simulink model "rl_distillation"  (R2022b)
settings: Solver=ode45  StartTime=0.0  StopTime=Tf  RelTol=1e-3  EnableMultiTasking=on
model workspace (MAT data in the model file):
  DM0 = [1  0; 0  1]
  G = tf
  G.InputName_ = ["u1"; "u2"]
  G.OutputName_ = ["y1"; "y2"]
  G.IOSize_ = [2 2]
  G.Data_ = ltipack.tfdata
  G.Data_.num = {[0 87.8], [0 -86.4]; [0 108.2], [0 -109.6]}
  G.Data_.den = {[75 1], [75 1]; [75 1], [75 1]}
  G.Data_.Delay.Input = [0; 0]
  G.Data_.Delay.Output = [0; 0]
  G.Data_.Delay.IO = [0  0; 0  0]
  G.Data_.Ts = 0
undefined symbols (not defined in the file or in its folder): random_refs_table, Tf
libraries: slpidlib x2, cstblocks x1, rllib x1
settings Model: Creator=The MathWorks, Inc.  LastModifiedBy=enes
settings SolverCC: AlgebraicLoopSolver=TrustRegion  MaxZcPerStep=1
settings DataIOCC: LimitDataPoints=on  SaveFormat=Array  ReturnWorkspaceOutputs=off
settings OptimizationCC: ExpressionDepthLimit=2147483647  LifeSpan=inf
settings DebuggingCC: UnderspecifiedInitializationDetection=Classic  MergeDetectMultiDrivingBlocksExec=none  FcnCallInpInsideContextMsg=warning  UnconnectedInputMsg=warning  UnconnectedOutputMsg=warning  UnconnectedLineMsg=warning  StateNameClashWarn=warning  SFUnexpectedBacktrackingDiag=warning  SFNoUnconditionalDefaultTransitionDiag=warning  SFMachineParentedDataDiag=warning  ArithmeticOperatorsInVariantConditions=warning
settings HardwareCC: ProdBitPerPointer=32  ProdBitPerSizeT=32  ProdBitPerPtrDiffT=32  ProdLargestAtomicFloat=None  ProdIntDivRoundTo=Undefined  ProdEndianess=Unspecified  ProdWordSize=32  ProdHWDeviceType=32-bit Generic
settings ModelReferenceCC: EnableRefExpFcnMdlSchedulingChecks=on  PropagateSignalLabelsOutOfModel=off
settings SFSimCC: SimUseLocalCustomCode=off  CustomCodeUndefinedFunction=UseInterfaceOnly
settings RTWCC: RTWUseLocalCustomCode=off  DLArmComputeVersion=19.05
settings CodeAppCC: StateflowObjectComments=on
settings GRTTargetCC: TargetLangStandard=C89/C90 (ANSI)  CombineOutputUpdateFcns=off  GRTInterface=on
settings ConfigComp: CovMetricSettings=dw  CovSaveCumulativeToWorkspaceVar=on  CovSaveSingleToWorkspaceVar=on  CovExternalEMLEnable=off  CovSFcnEnable=off

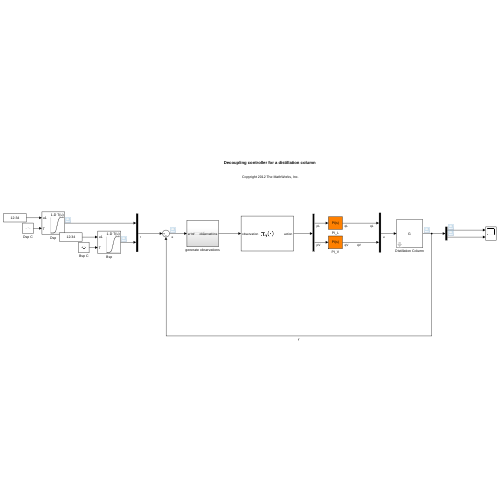
[thumbnail: Simulink's stored preview of the top-level diagram]
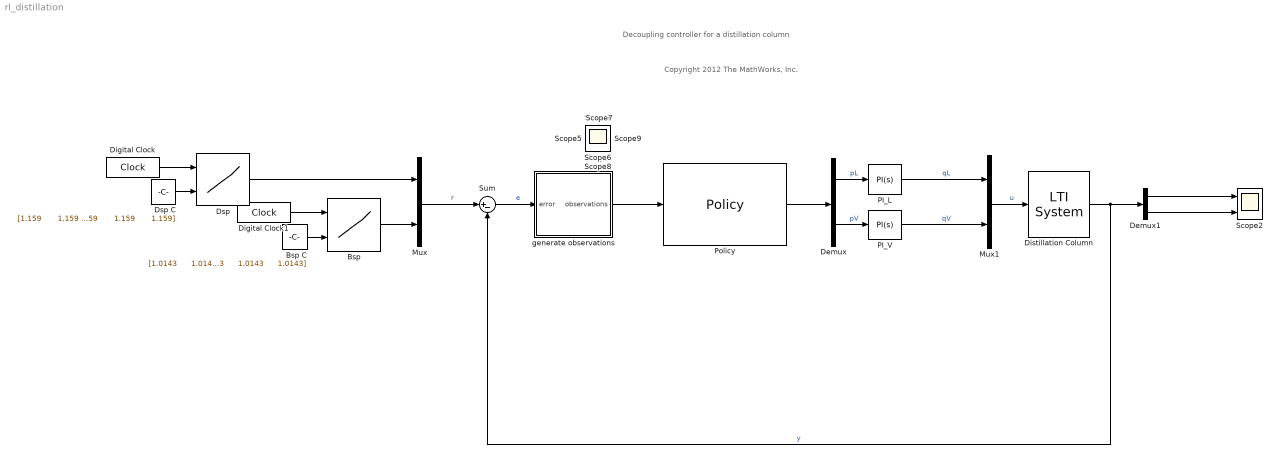
== system rl_distillation ==
  note: Copyright 2012 The MathWorks, Inc.
  note: Decoupling controller for a distillation column
  Bsp : Lookup_n-D  NumberOfTableDimensions=1  BreakpointsForDimension1=[1:Tf]  TableSource=Input port  Table=random_refs_table  InternalRulePriority=Speed  RndMeth=Simplest
      settings: InputPortMap=u0,p221
  Bsp C : Constant  Value="[1.0143      1.0143      1.0143      1.0143      1.0143      1.0143      1.0143      1.0143      1.0143      1.0143      1.0143      1.0143      1.0143      1.0143      1.0143      1.0143      1.0143      1.0143      1.0143      1.0143      1.0143      1.0143      1.0143      1.0143      1.0143      1.0143      1.0143      1.0143      1.0143      1.0143      1.0143      1.0143      1.0143      1.0143      1.0143      1.0143      1.0143      1.0143      1.0143      1.0143      1.0143      1.0143      1.0143      1.0143      1.0143      1.0143      1.0143      1.0143      1.0143      1.0143      1.0143      1.0143      1.0143      1.0143      1.0143      1.0143      1.0143      1.0143      1.0143      1.0143      1.0143      1.0143      1.0143      1.0143      1.0143      1.0143      1.0143      1.0143      1.0143      1.0143      1.0143      1.0143      1.0143      1.0143      1.0143]"
  Demux : Demux  Outputs=2
  Demux1 : Demux  Outputs=2
  Digital Clock : DigitalClock
  Digital Clock1 : DigitalClock
  Distillation Column : cstblocks/LTI System  sys=G  IC=[]
  Dsp : Lookup_n-D  NumberOfTableDimensions=1  BreakpointsForDimension1=[1:Tf]  TableSource=Input port  Table=random_refs_table  InternalRulePriority=Speed  RndMeth=Simplest
      settings: InputPortMap=u0,p221
  Dsp C : Constant  Value="[1.159       1.159       1.159       1.159       1.159       1.159       1.159       1.159       1.159       1.159       1.159       1.159       1.159       1.159       1.159       1.159       1.159       1.159       1.159       1.159       1.159       1.159       1.159       1.159       1.159       1.159       1.159       1.159       1.159       1.159       1.159       1.159       1.159       1.159       1.159       1.159       1.159       1.159       1.159       1.159       1.159       1.159       1.159       1.159       1.159       1.159       1.159       1.159       1.159       1.159       1.159       1.159       1.159       1.159       1.159       1.159       1.159       1.159       1.159       1.159       1.159       1.159       1.159       1.159       1.159       1.159       1.159       1.159       1.159       1.159       1.159       1.159       1.159       1.159       1.159]"
  Mux : Mux  Inputs=2
  Mux1 : Mux  Inputs=2
  PI_L : slpidlib/PID Controller  Controller=PI  Form=Parallel  TimeDomain=Continuous-time  UseExternalTs=off  SampleTime=-1  IntegratorMethod=Forward Euler  FilterMethod=Forward Euler  ControllerParametersSource=internal  P=16.3  I=2.18  UseKiTs=off  D=0  N=100  UseFilter=on  TunerSelectOption=Transfer Function Based (PID Tuner App)  InitialConditionSource=internal  InitialConditionForIntegrator=0  InitialConditionForFilter=0  DifferentiatorICPrevScaledInput=0  ExternalReset=none  TrackingMode=off  Kt=1  LimitOutput=off  SatLimitsSource=internal  UpperSaturationLimit=inf  LowerSaturationLimit=-inf  LinearizeAsGain=off  AntiWindupMode=none  Kb=1  LimitIntegrator=off  UpperIntegratorSaturationLimit=inf  LowerIntegratorSaturationLimit=-inf  POutMin=[]  POutMax=[]  IOutMin=[]  IOutMax=[]  DOutMin=[]  DOutMax=[]  NOutMin=[]  NOutMax=[]  SumOutMin=[]  SumOutMax=[]  SaturationOutMin=[]  SaturationOutMax=[]  PParamMin=[]  PParamMax=[]  IParamMin=[]  IParamMax=[]  DParamMin=[]  DParamMax=[]  NParamMin=[]  NParamMax=[]  KbParamMin=[]  KbParamMax=[]  KtParamMin=[]  KtParamMax=[]  KbOutMin=[]  KbOutMax=[]  KtOutMin=[]  KtOutMax=[]  IntegratorOutMin=[]  IntegratorOutMax=[]  FilterOutMin=[]  FilterOutMax=[]  SumI1OutMin=[]  SumI1OutMax=[]  SumI2OutMin=[]  SumI2OutMax=[]  SumI3OutMin=[]  SumI3OutMax=[]  SumI4OutMin=[]  SumI4OutMax=[]  SumDOutMin=[]  SumDOutMax=[]  DifferentiatorOutMin=[]  DifferentiatorOutMax=[]  FilterDiffOutCoefMin=[]  FilterDiffOutCoefMax=[]  ReciprocalOutMin=[]  ReciprocalOutMax=[]  SumDenOutMin=[]  SumDenOutMax=[]  SumNumOutMin=[]  SumNumOutMax=[]  DivideOutMin=[]  DivideOutMax=[]  UdiffTsProdOutMin=[]  UdiffTsProdOutMax=[]  NTsProdOutMin=[]  NTsProdOutMax=[]  UintegralTsProdOutMin=[]  UintegralTsProdOutMax=[]  UngainTsProdOutMin=[]  UngainTsProdOutMax=[]  ClampingZeroOutDataTypeStr=Inherit: Inherit via back propagation  ClampingZeroOutMin=[]  ClampingZeroOutMax=[]  FilterDenConstantOutDataTypeStr=Inherit: Inherit via back propagation  FilterDenConstantOutMin=[]  FilterDenConstantOutMax=[]  PCopyOutDataTypeStr=Inherit: Inherit via back propagation  PCopyOutMin=[]  PCopyOutMax=[]  NCopyOutDataTypeStr=Inherit: Inherit via back propagation  NCopyOutMin=[]  NCopyOutMax=[]  IntegratorContinuousStateAttributes=''  IntegratorStateMustResolveToSignalObject=off  IntegratorRTWStateStorageClass=Auto  FilterContinuousStateAttributes=''  FilterStateMustResolveToSignalObject=off  FilterRTWStateStorageClass=Auto  ParallelPVariant=InternalParameters  IdealPVariant=Disabled  IVariant=InternalParameters  DVariant=Disabled  IntegratorVariant=Continuous  SatVariant=Disabled  AWVariant=Passthrough  PCopyVariant=Disabled  TRVariant=Disabled  FdbkBlocksVariant=Forward  IdealPFdbkVariant=Disabled  SatFdbkVariant=Disabled  DerivativeFilterVariant=Disabled  NVariant=Disabled  NCopyVariant=Disabled_SignalSpec  FilterICVariant=Disabled  IntegratorICVariant=InternalICs  ExternalResetVariant=Disabled  TRSumVariant=Passthrough  SumFdbkVariant=Disabled  SumVariant=Sum_PI  TsampFilterVariant=InternalTs  TsampNgainVariant=Passthrough  TsampIntegralVariant=Passthrough  ExternalSaturationOutDataTypeStr=Inherit: Same as second input
  PI_V : slpidlib/PID Controller  Controller=PI  Form=Parallel  TimeDomain=Continuous-time  UseExternalTs=off  SampleTime=-1  IntegratorMethod=Forward Euler  FilterMethod=Forward Euler  ControllerParametersSource=internal  P=13.1  I=1.76  UseKiTs=off  D=0  N=100  UseFilter=on  TunerSelectOption=Transfer Function Based (PID Tuner App)  InitialConditionSource=internal  InitialConditionForIntegrator=0  InitialConditionForFilter=0  DifferentiatorICPrevScaledInput=0  ExternalReset=none  TrackingMode=off  Kt=1  LimitOutput=off  SatLimitsSource=internal  UpperSaturationLimit=inf  LowerSaturationLimit=-inf  LinearizeAsGain=off  AntiWindupMode=none  Kb=1  LimitIntegrator=off  UpperIntegratorSaturationLimit=inf  LowerIntegratorSaturationLimit=-inf  POutMin=[]  POutMax=[]  IOutMin=[]  IOutMax=[]  DOutMin=[]  DOutMax=[]  NOutMin=[]  NOutMax=[]  SumOutMin=[]  SumOutMax=[]  SaturationOutMin=[]  SaturationOutMax=[]  PParamMin=[]  PParamMax=[]  IParamMin=[]  IParamMax=[]  DParamMin=[]  DParamMax=[]  NParamMin=[]  NParamMax=[]  KbParamMin=[]  KbParamMax=[]  KtParamMin=[]  KtParamMax=[]  KbOutMin=[]  KbOutMax=[]  KtOutMin=[]  KtOutMax=[]  IntegratorOutMin=[]  IntegratorOutMax=[]  FilterOutMin=[]  FilterOutMax=[]  SumI1OutMin=[]  SumI1OutMax=[]  SumI2OutMin=[]  SumI2OutMax=[]  SumI3OutMin=[]  SumI3OutMax=[]  SumI4OutMin=[]  SumI4OutMax=[]  SumDOutMin=[]  SumDOutMax=[]  DifferentiatorOutMin=[]  DifferentiatorOutMax=[]  FilterDiffOutCoefMin=[]  FilterDiffOutCoefMax=[]  ReciprocalOutMin=[]  ReciprocalOutMax=[]  SumDenOutMin=[]  SumDenOutMax=[]  SumNumOutMin=[]  SumNumOutMax=[]  DivideOutMin=[]  DivideOutMax=[]  UdiffTsProdOutMin=[]  UdiffTsProdOutMax=[]  NTsProdOutMin=[]  NTsProdOutMax=[]  UintegralTsProdOutMin=[]  UintegralTsProdOutMax=[]  UngainTsProdOutMin=[]  UngainTsProdOutMax=[]  ClampingZeroOutDataTypeStr=Inherit: Inherit via back propagation  ClampingZeroOutMin=[]  ClampingZeroOutMax=[]  FilterDenConstantOutDataTypeStr=Inherit: Inherit via back propagation  FilterDenConstantOutMin=[]  FilterDenConstantOutMax=[]  PCopyOutDataTypeStr=Inherit: Inherit via back propagation  PCopyOutMin=[]  PCopyOutMax=[]  NCopyOutDataTypeStr=Inherit: Inherit via back propagation  NCopyOutMin=[]  NCopyOutMax=[]  IntegratorContinuousStateAttributes=''  IntegratorStateMustResolveToSignalObject=off  IntegratorRTWStateStorageClass=Auto  FilterContinuousStateAttributes=''  FilterStateMustResolveToSignalObject=off  FilterRTWStateStorageClass=Auto  ParallelPVariant=InternalParameters  IdealPVariant=Disabled  IVariant=InternalParameters  DVariant=Disabled  IntegratorVariant=Continuous  SatVariant=Disabled  AWVariant=Passthrough  PCopyVariant=Disabled  TRVariant=Disabled  FdbkBlocksVariant=Forward  IdealPFdbkVariant=Disabled  SatFdbkVariant=Disabled  DerivativeFilterVariant=Disabled  NVariant=Disabled  NCopyVariant=Disabled_SignalSpec  FilterICVariant=Disabled  IntegratorICVariant=InternalICs  ExternalResetVariant=Disabled  TRSumVariant=Passthrough  SumFdbkVariant=Disabled  SumVariant=Sum_PI  TsampFilterVariant=InternalTs  TsampNgainVariant=Passthrough  TsampIntegralVariant=Passthrough  ExternalSaturationOutDataTypeStr=Inherit: Same as second input
  Policy : rllib/Policy  MATFile=blockAgentData.mat  SimUsingCodegen=off
  Scope2 : Scope  NumInputPorts=2
  Sum : Sum  Inputs=|+-
  generate observations : Subsystem
  Scope{,1,3..9} (9 alike) : Scope
  wires:
  Dsp/1 -> Mux/1
  Bsp/1 -> Mux/2
  Mux/1 -> Sum/1  "r"
  Demux/1 -> PI_L/1  "pL"
  Demux/2 -> PI_V/1  "pV"
  Distillation Column/1 -> Sum/2, Demux1/1  "y"
  Mux1/1 -> Distillation Column/1  "u"
  PI_V/1 -> Mux1/2  "qV"
  PI_L/1 -> Mux1/1  "qL"
  Policy/1 -> Demux/1
  generate observations/1(observations) -> Policy/1
  Sum/1 -> generate observations/1(error)  "e"
  Demux1/1 -> Scope2/1
  Demux1/2 -> Scope2/2
  Dsp C/1 -> Dsp/2
  Digital Clock/1 -> Dsp/1
  Bsp C/1 -> Bsp/2
  Digital Clock1/1 -> Bsp/1

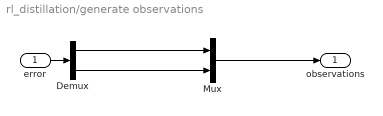
== system rl_distillation/generate observations ==
  error : Inport
  Demux : Demux  Outputs=2
  Mux : Mux  Inputs=2
  observations : Outport  VectorParamsAs1DForOutWhenUnconnected=off
  wires:
  Mux/1 -> observations/1
  error/1 -> Demux/1
  Demux/1 -> Mux/1
  Demux/2 -> Mux/2
